simulink model "basicmodel"  (R2018a)
settings: Solver=ode3  StartTime=0.0  StopTime=100  FixedStep=0.1  RelTol=1e-3
InitFcn:
  | data
undefined symbols (not defined in the file or in its folder): sigbuilder_block
libraries: simulink x8
settings Model: Creator=dhruv  LastModifiedBy=dhruv

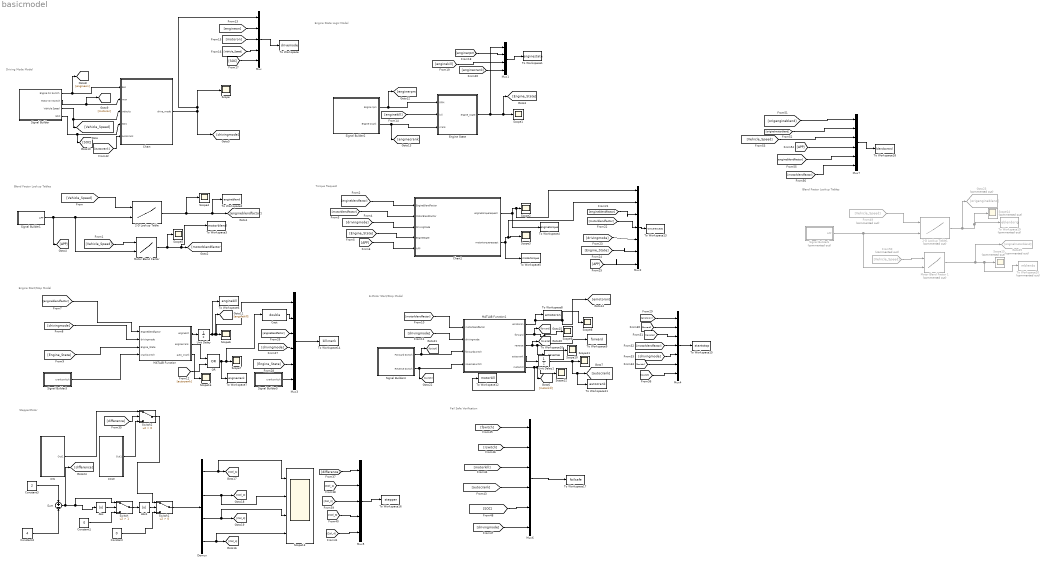
== system basicmodel ==
  note: Fail Safe Verification
  note: E-Motor Start/Stop Model
  note: Engine Start/Stop Model
  note: Torque Request
  note: Engine State Logic Model
  note: Blend Factor Lookup Tables
  note: Driving Mode Model
  note: StepperMotor
  note: Blend Factor Lookup Tables
  2-D Lookup Table : Lookup_n-D  InitFcn=data  BreakpointsForDimension1=Engine_Blend_Factor(2:end,1)  BreakpointsForDimension2=Engine_Blend_Factor(1,2:end)  Table=Engine_Blend_Factor(2:end,2:end)  InternalRulePriority=Speed  RndMeth=Simplest  InputSameDT=on
  2-D Lookup Table1 : Lookup_n-D  Commented=on  InitFcn=data  BreakpointsForDimension1=Engine_Blend_Factoro(2:end,1)  BreakpointsForDimension2=Engine_Blend_Factoro(1,2:end)  Table=Engine_Blend_Factoro(2:end,2:end)  InternalRulePriority=Speed  RndMeth=Simplest  InputSameDT=on
  Abs : Abs
  Abs1 : Abs
  CCW : Subsystem
  CW : Subsystem
  Cast : DataTypeConversion  OutDataTypeStr=double
  Chart : Stateflow chart  TreatAsAtomicUnit=on
  Chart1 : Stateflow chart  TreatAsAtomicUnit=on
  Constant : Constant  Value=0
  Constant1 : Constant  Value=0
  Constant3 : Constant  Value=2
  Constant4 : Constant  Value=4
  Demux : Demux
  "Engine State " : Stateflow chart  TreatAsAtomicUnit=on
  From49 : From  Commented=on  GotoTag=Vehicle_Speed
  From50 : From  Commented=on  GotoTag=Vehicle_Speed
  Goto23 : Goto  Commented=on  GotoTag=origengineblend
  Goto25 : Goto  Commented=on  GotoTag=originalmotorblend
  MATLAB Function : MATLAB Function  TreatAsAtomicUnit=on
  MATLAB Function1 : MATLAB Function  TreatAsAtomicUnit=on
  "Motor Blend Factor " : Lookup_n-D  BreakpointsForDimension1=Motor_Blend_Factor(2:end,1)  BreakpointsForDimension2=Motor_Blend_Factor(1,2:end)  Table=Motor_Blend_Factor(2:end,2:end)  InternalRulePriority=Speed  RndMeth=Simplest  InputSameDT=on
  Motor Blend Factor 1 : Lookup_n-D  Commented=on  BreakpointsForDimension1=Motor_Blend_Factoro(2:end,1)  BreakpointsForDimension2=Motor_Blend_Factoro(1,2:end)  Table=Motor_Blend_Factoro(2:end,2:end)  InternalRulePriority=Speed  RndMeth=Simplest  InputSameDT=on
  Mux : Mux  Inputs=5
  Mux1 : Mux
  Mux2 : Mux  Inputs=7
  Mux3 : Mux  Inputs=6
  Mux4 : Mux  Inputs=7
  Mux5 : Mux  Inputs=5
  Mux6 : Mux  Inputs=6
  Mux7 : Mux  Inputs=6
  OR : Logic  Operator=OR  IconShape=distinctive  AllPortsSameDT=off  OutDataTypeStr=boolean
  Scope{,1..12,16} (14 alike) : Scope
  Scope13 : Scope  NumInputPorts=4
  Scope14 : Scope  Commented=on
  Scope15 : Scope  Commented=on
  Signal Builder : Subsystem  Tag=STV Subsys  LoadFcn=sigbuilder_block('load');  StartFcn=sigbuilder_block('start');  StopFcn=sigbuilder_block('stop');  ClipboardFcn=sigbuilder_block('clipboard');  mask(Sigbuilder block){tuvar=[0:10]}
      mask help: Simulink:masks:SigbuilderBlock_MD
      mask init:
      | if ~strcmp(get_param(bdroot(gcbh),'SimulationStatus'),'stopped') tuvar = sigbuilder_block('maskInit'); end
      settings: CopyFcn=sigbuilder_block('copy');  DeleteFcn=sigbuilder_block('delete');  ModelCloseFcn=sigbuilder_block('modelClose');  PreSaveFcn=sigbuilder_block('preSave');  PauseFcn=sigbuilder_block('pause');  ContinueFcn=sigbuilder_block('continue');  NameChangeFcn=sigbuilder_block('namechange');  OpenFcn=sigbuilder_block('open',[5.5 30 949 418 ]);  CloseFcn=sigbuilder_block('close');
      mask Display: plot(0, 0, 100, 100,[2, 2, 32, 32, 2], [68, 8, 8, 68, 68],[32, 2], [38, 38], [32, 19, 2],[53, 60, 44], [32, 17, 17, 2],[16, 16, 31, 31]);txt = getActiveGroup(gcbh);text(2, 100, txt,'verticalAlignment', 'top');
  Signal Builder1 : Subsystem  Tag=STV Subsys  LoadFcn=sigbuilder_block('load');  StartFcn=sigbuilder_block('start');  StopFcn=sigbuilder_block('stop');  ClipboardFcn=sigbuilder_block('clipboard');  mask(Sigbuilder block){tuvar=[0:10]}
      mask help: Simulink:masks:SigbuilderBlock_MD
      mask init:
      | if ~strcmp(get_param(bdroot(gcbh),'SimulationStatus'),'stopped') tuvar = sigbuilder_block('maskInit'); end
      settings: CopyFcn=sigbuilder_block('copy');  DeleteFcn=sigbuilder_block('delete');  ModelCloseFcn=sigbuilder_block('modelClose');  PreSaveFcn=sigbuilder_block('preSave');  PauseFcn=sigbuilder_block('pause');  ContinueFcn=sigbuilder_block('continue');  NameChangeFcn=sigbuilder_block('namechange');  OpenFcn=sigbuilder_block('open',[267 99 550.5 362.5 ]);  CloseFcn=sigbuilder_block('close');
      mask Display: plot(0, 0, 100, 100,[2, 2, 32, 32, 2], [68, 8, 8, 68, 68],[32, 2], [38, 38], [32, 19, 2],[53, 60, 44], [32, 17, 17, 2],[16, 16, 31, 31]);txt = getActiveGroup(gcbh);text(2, 100, txt,'verticalAlignment', 'top');
  Signal Builder2 : Subsystem  Tag=STV Subsys  LoadFcn=sigbuilder_block('load');  StartFcn=sigbuilder_block('start');  StopFcn=sigbuilder_block('stop');  ClipboardFcn=sigbuilder_block('clipboard');  mask(Sigbuilder block){tuvar=[0:10]}
      mask help: Simulink:masks:SigbuilderBlock_MD
      mask init:
      | if ~strcmp(get_param(bdroot(gcbh),'SimulationStatus'),'stopped') tuvar = sigbuilder_block('maskInit'); end
      settings: CopyFcn=sigbuilder_block('copy');  DeleteFcn=sigbuilder_block('delete');  ModelCloseFcn=sigbuilder_block('modelClose');  PreSaveFcn=sigbuilder_block('preSave');  PauseFcn=sigbuilder_block('pause');  ContinueFcn=sigbuilder_block('continue');  NameChangeFcn=sigbuilder_block('namechange');  OpenFcn=sigbuilder_block('open',[5.5 30 949 418 ]);  CloseFcn=sigbuilder_block('close');
      mask Display: plot(0, 0, 100, 100,[2, 2, 32, 32, 2], [68, 8, 8, 68, 68],[32, 2], [38, 38], [32, 19, 2],[53, 60, 44], [32, 17, 17, 2],[16, 16, 31, 31]);txt = getActiveGroup(gcbh);text(2, 100, txt,'verticalAlignment', 'top');
  Signal Builder3 : Subsystem  Tag=STV Subsys  LoadFcn=sigbuilder_block('load');  StartFcn=sigbuilder_block('start');  StopFcn=sigbuilder_block('stop');  ClipboardFcn=sigbuilder_block('clipboard');  mask(Sigbuilder block){tuvar=[0:10]}
      mask help: Simulink:masks:SigbuilderBlock_MD
      mask init:
      | if ~strcmp(get_param(bdroot(gcbh),'SimulationStatus'),'stopped') tuvar = sigbuilder_block('maskInit'); end
      settings: CopyFcn=sigbuilder_block('copy');  DeleteFcn=sigbuilder_block('delete');  ModelCloseFcn=sigbuilder_block('modelClose');  PreSaveFcn=sigbuilder_block('preSave');  PauseFcn=sigbuilder_block('pause');  ContinueFcn=sigbuilder_block('continue');  NameChangeFcn=sigbuilder_block('namechange');  OpenFcn=sigbuilder_block('open',[404 117.5 550.5 362.5 ]);  CloseFcn=sigbuilder_block('close');
      mask Display: plot(0, 0, 100, 100,[2, 2, 32, 32, 2], [68, 8, 8, 68, 68],[32, 2], [38, 38], [32, 19, 2],[53, 60, 44], [32, 17, 17, 2],[16, 16, 31, 31]);txt = getActiveGroup(gcbh);text(2, 100, txt,'verticalAlignment', 'top');
  Signal Builder4 : Subsystem  Tag=STV Subsys  LoadFcn=sigbuilder_block('load');  StartFcn=sigbuilder_block('start');  StopFcn=sigbuilder_block('stop');  ClipboardFcn=sigbuilder_block('clipboard');  mask(Sigbuilder block){tuvar=[0:10]}
      mask help: Simulink:masks:SigbuilderBlock_MD
      mask init:
      | if ~strcmp(get_param(bdroot(gcbh),'SimulationStatus'),'stopped') tuvar = sigbuilder_block('maskInit'); end
      settings: CopyFcn=sigbuilder_block('copy');  DeleteFcn=sigbuilder_block('delete');  ModelCloseFcn=sigbuilder_block('modelClose');  PreSaveFcn=sigbuilder_block('preSave');  PauseFcn=sigbuilder_block('pause');  ContinueFcn=sigbuilder_block('continue');  NameChangeFcn=sigbuilder_block('namechange');  OpenFcn=sigbuilder_block('open',[404 117.5 550.5 362.5 ]);  CloseFcn=sigbuilder_block('close');
      mask Display: plot(0, 0, 100, 100,[2, 2, 32, 32, 2], [68, 8, 8, 68, 68],[32, 2], [38, 38], [32, 19, 2],[53, 60, 44], [32, 17, 17, 2],[16, 16, 31, 31]);txt = getActiveGroup(gcbh);text(2, 100, txt,'verticalAlignment', 'top');
  Signal Builder5 : Subsystem  Tag=STV Subsys  LoadFcn=sigbuilder_block('load');  StartFcn=sigbuilder_block('start');  StopFcn=sigbuilder_block('stop');  ClipboardFcn=sigbuilder_block('clipboard');  mask(Sigbuilder block){tuvar=[0:10]}
      mask help: Simulink:masks:SigbuilderBlock_MD
      mask init:
      | if ~strcmp(get_param(bdroot(gcbh),'SimulationStatus'),'stopped') tuvar = sigbuilder_block('maskInit'); end
      settings: CopyFcn=sigbuilder_block('copy');  DeleteFcn=sigbuilder_block('delete');  ModelCloseFcn=sigbuilder_block('modelClose');  PreSaveFcn=sigbuilder_block('preSave');  PauseFcn=sigbuilder_block('pause');  ContinueFcn=sigbuilder_block('continue');  NameChangeFcn=sigbuilder_block('namechange');  OpenFcn=sigbuilder_block('open',[404 117.5 550.5 362.5 ]);  CloseFcn=sigbuilder_block('close');
      mask Display: plot(0, 0, 100, 100,[2, 2, 32, 32, 2], [68, 8, 8, 68, 68],[32, 2], [38, 38], [32, 19, 2],[53, 60, 44], [32, 17, 17, 2],[16, 16, 31, 31]);txt = getActiveGroup(gcbh);text(2, 100, txt,'verticalAlignment', 'top');
  Signal Builder6 : Subsystem  Tag=STV Subsys  Commented=on  LoadFcn=sigbuilder_block('load');  StartFcn=sigbuilder_block('start');  StopFcn=sigbuilder_block('stop');  ClipboardFcn=sigbuilder_block('clipboard');  mask(Sigbuilder block){tuvar=[0:10]}
      mask help: Simulink:masks:SigbuilderBlock_MD
      mask init:
      | if ~strcmp(get_param(bdroot(gcbh),'SimulationStatus'),'stopped') tuvar = sigbuilder_block('maskInit'); end
      settings: CopyFcn=sigbuilder_block('copy');  DeleteFcn=sigbuilder_block('delete');  ModelCloseFcn=sigbuilder_block('modelClose');  PreSaveFcn=sigbuilder_block('preSave');  PauseFcn=sigbuilder_block('pause');  ContinueFcn=sigbuilder_block('continue');  NameChangeFcn=sigbuilder_block('namechange');  OpenFcn=sigbuilder_block('open',[267 99 550.5 362.5 ]);  CloseFcn=sigbuilder_block('close');
      mask Display: plot(0, 0, 100, 100,[2, 2, 32, 32, 2], [68, 8, 8, 68, 68],[32, 2], [38, 38], [32, 19, 2],[53, 60, 44], [32, 17, 17, 2],[16, 16, 31, 31]);txt = getActiveGroup(gcbh);text(2, 100, txt,'verticalAlignment', 'top');
  Sum : Sum  Inputs=+-
  Switch : Switch  Criteria=u2 > Threshold  Threshold=1
  Switch1 : Switch  Criteria=u2 > Threshold
  Switch2 : Switch  Criteria=u2 > Threshold
  To Workspace : ToWorkspace  VariableName=drivemode  SaveFormat=Timeseries  SampleTime=-1
  To Workspace1 : ToWorkspace  VariableName=enginestate  SaveFormat=Timeseries  SampleTime=-1
  To Workspace10 : ToWorkspace  VariableName=reverse  SaveFormat=Timeseries  SampleTime=-1
  To Workspace11 : ToWorkspace  VariableName=autocrank  SaveFormat=Timeseries  SampleTime=-1
  To Workspace12 : ToWorkspace  VariableName=motorkill  SaveFormat=Timeseries  SampleTime=-1
  To Workspace13 : ToWorkspace  VariableName=torquerequests  SaveFormat=Timeseries  SampleTime=-1
  To Workspace14 : ToWorkspace  VariableName=killcrank  SaveFormat=Timeseries  SampleTime=-1
  To Workspace15 : ToWorkspace  VariableName=startstop  SaveFormat=Timeseries  SampleTime=-1
  To Workspace16 : ToWorkspace  VariableName=stepper  SaveFormat=Timeseries  SampleTime=-1
  To Workspace17 : ToWorkspace  VariableName=failsafe  SaveFormat=Timeseries  SampleTime=-1
  To Workspace18 : ToWorkspace  VariableName=blendcontrol  SaveFormat=Timeseries  SampleTime=-1
  To Workspace19 : ToWorkspace  Commented=on  VariableName=eblendorig  SaveFormat=Timeseries  SampleTime=-1
  To Workspace2 : ToWorkspace  VariableName=engineblend  SaveFormat=Timeseries  SampleTime=-1
  To Workspace20 : ToWorkspace  Commented=on  VariableName=mblendo  SaveFormat=Timeseries  SampleTime=-1
  To Workspace3 : ToWorkspace  VariableName=motorblend  SaveFormat=Timeseries  SampleTime=-1
  To Workspace4 : ToWorkspace  VariableName=enginetorque  SaveFormat=Timeseries  SampleTime=-1
  To Workspace5 : ToWorkspace  VariableName=motortorque  SaveFormat=Timeseries  SampleTime=-1
  To Workspace6 : ToWorkspace  VariableName=enginekill  SaveFormat=Timeseries  SampleTime=-1
  To Workspace7 : ToWorkspace  VariableName=enginecrank  SaveFormat=Timeseries  SampleTime=-1
  To Workspace8 : ToWorkspace  VariableName=emotoron  SaveFormat=Timeseries  SampleTime=-1
  To Workspace9 : ToWorkspace  VariableName=forward  SaveFormat=Timeseries  SampleTime=-1
  Unit Delay : UnitDelay  SampleTime=-1
  Unit Delay1 : UnitDelay  SampleTime=-1
  wires:
  Signal Builder/2(Motor On Switch) -> [motoron], Chart/2(mon)
  Signal Builder/1(Engine On Switch) -> [engineon], Chart/1(Eon)
  Signal Builder/3(Vehicle Speed) -> [Vehicle_Speed], Chart/3(velocity)
  Signal Builder1/1(APP) -> [APP], "Motor Blend Factor "/2, 2-D Lookup Table/2
  [Vehicle_Speed] -> 2-D Lookup Table/1
  [Vehicle_Speed] -> "Motor Blend Factor "/1
  2-D Lookup Table/1 -> Scope4/1, To Workspace2/1, [engineblendfactor]
  "Motor Blend Factor "/1 -> Scope5/1, To Workspace3/1, [motorblendfactor]
  Chart/1(drive_mode) -> Mux/1, Scope/1, [drivingmode]
  Signal Builder2/1(Engine rpm) -> [enginerpm], "Engine State "/1(RPM)
  [engineblendfactor] -> Chart1/1(EngineBlendFactor)
  [motorblendfactor] -> Chart1/2(MotorBlendFactor)
  [drivingmode] -> Chart1/3(DrivingMode)
  [Engine_State] -> Chart1/4(EngineState)
  [APP] -> Chart1/5(APP)
  Chart1/1(enginetorquerequest) -> Mux2/1, Scope2/1, To Workspace4/1
  Chart1/2(motortorquerequest) -> Mux2/2, Scope3/1, To Workspace5/1
  [engineblendfactor] -> MATLAB Function/1(engineblendfactor)
  [drivingmode] -> MATLAB Function/2(drivingmode)
  [Engine_State] -> MATLAB Function/3(Engine_State)
  Signal Builder3/1(crankswitch) -> MATLAB Function/4(crankswitch)
  MATLAB Function/2(enginecrank) -> OR/1
  [motorblendfactor] -> MATLAB Function1/1(motorblendfactor)
  [drivingmode] -> MATLAB Function1/2(drivingmode)
  Signal Builder4/1(Forward Switch) -> [fswitch], MATLAB Function1/3(forwardswitch)
  Signal Builder4/2(Reverse Switch) -> [rswitch], MATLAB Function1/4(reverseswitch)
  MATLAB Function1/1(emotoron) -> To Workspace8/1, [emotoron], Scope8/1
  MATLAB Function1/3(reverse) -> [reverse], To Workspace10/1, Scope10/1
  [enginekill] -> "Engine State "/2(kill)
  MATLAB Function/1(enginekill) -> Unit Delay/1
  "Engine State "/1(engine_state) -> Mux1/1, [Engine_State], Scope1/1
  Unit Delay/1 -> To Workspace6/1, [enginekill], Mux3/1, Scope6/1
  MATLAB Function1/2(forward) -> [forward], To Workspace9/1, Scope9/1
  MATLAB Function1/4(autocrank) -> Unit Delay1/1
  MATLAB Function1/5(motorkill) -> To Workspace12/1, [motorkill], Scope12/1
  [difference] -> Switch2/2
  CCW/1(Out1) -> Switch2/3
  CW/1(Out1) -> Switch2/1
  Constant3/1 -> Sum/1
  Demux/4 -> Scope13/4, [Coil_4]
  Constant4/1 -> Sum/2
  Demux/1 -> Scope13/1, [Coil_1]
  Demux/2 -> Scope13/2, [Coil_2]
  Sum/1 -> [difference], Switch/1, Abs/1
  Demux/3 -> Scope13/3, [Coil_3]
  Abs/1 -> Switch/2
  [autocrank] -> OR/2
  OR/1 -> To Workspace7/1, Cast/1, Scope7/1
  Switch/1 -> Abs1/1
  Switch2/1 -> Switch1/1
  Constant/1 -> Switch1/3
  Switch1/1 -> Demux/1
  Constant1/1 -> Switch/3
  Abs1/1 -> Switch1/2
  Signal Builder/4(SOC) -> [SOC], Chart/4(SOC)
  [engineon] -> Mux/2
  [motoron] -> Mux/3
  [Vehicle_Speed] -> Mux/4
  [SOC] -> Mux/5
  Mux/1 -> To Workspace/1
  Signal Builder2/2(Engine Crank) -> [enginecrank], "Engine State "/3(crank)
  Mux1/1 -> To Workspace1/1
  [enginerpm] -> Mux1/2
  [enginekill] -> Mux1/3
  [enginecrank] -> Mux1/4
  [engineblendfactor] -> Mux2/3
  [motorblendfactor] -> Mux2/4
  [drivingmode] -> Mux2/5
  [Engine_State] -> Mux2/6
  [APP] -> Mux2/7
  Mux2/1 -> To Workspace13/1
  [engineblendfactor] -> Mux3/3
  [drivingmode] -> Mux3/4
  [Engine_State] -> Mux3/5
  Signal Builder5/1(crankswitch) -> Mux3/6
  Mux3/1 -> To Workspace14/1
  [emotoron] -> Mux4/1
  [forward] -> Mux4/2
  [reverse] -> Mux4/3
  [motorblendfactor] -> Mux4/4
  [drivingmode] -> Mux4/5
  [fswitch] -> Mux4/6
  [rswitch] -> Mux4/7
  Mux4/1 -> To Workspace15/1
  [difference] -> Mux5/1
  [Coil_1] -> Mux5/2
  [Coil_2] -> Mux5/3
  [Coil_3] -> Mux5/4
  [Coil_4] -> Mux5/5
  Mux5/1 -> To Workspace16/1
  Cast/1 -> Mux3/2
  [autocrank] -> Chart/5(autocrank)
  Unit Delay1/1 -> To Workspace11/1, [autocrank], Scope11/1
  [fswitch] -> Mux6/1
  [rswitch] -> Mux6/2
  [motorkill] -> Mux6/3
  [autocrank] -> Mux6/4
  [drivingmode] -> Mux6/6
  [SOC] -> Mux6/5
  Mux6/1 -> To Workspace17/1
  Signal Builder6/1(APP) -> Motor Blend Factor 1/2, 2-D Lookup Table1/2
  From49/1 -> 2-D Lookup Table1/1
  Motor Blend Factor 1/1 -> Goto25/1, To Workspace20/1, Scope15/1
  From50/1 -> Motor Blend Factor 1/1
  2-D Lookup Table1/1 -> Goto23/1, To Workspace19/1, Scope14/1
  [origengineblend] -> Mux7/1
  [originalmotorblend] -> Mux7/2
  [Vehicle_Speed] -> Mux7/3
  [APP] -> Mux7/4
  [engineblendfactor] -> Mux7/5
  [motorblendfactor] -> Mux7/6
  Mux7/1 -> To Workspace18/1
  MATLAB Function/3(auto_crank) -> Scope16/1

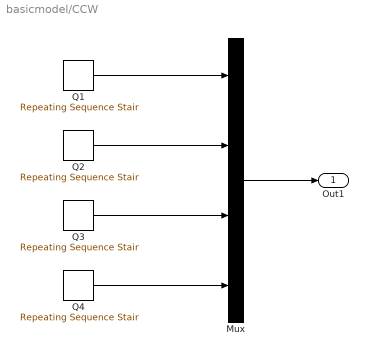
== system basicmodel/CCW ==
  Mux : Mux
  Q1 : simulink/Sources/Repeating Sequence Stair  OutValues=[1 0 0 0 0 0 1 1 1].'  tsamp=-1  OutMin=[]  OutMax=[]  OutDataTypeStr=double  OutputDataTypeScalingMode=double  OutDataType=fixdt(0,8)  ConRadixGroup=Best Precision: Vector-wise  OutScaling=2^-12
  Q2 : simulink/Sources/Repeating Sequence Stair  OutValues=[0 0 1 1 1 0 0 0 0].'  tsamp=-1  OutMin=[]  OutMax=[]  OutDataTypeStr=double  OutputDataTypeScalingMode=double  OutDataType=fixdt(0,8)  ConRadixGroup=Best Precision: Vector-wise  OutScaling=2^-12
  Q3 : simulink/Sources/Repeating Sequence Stair  OutValues=[1 1 1 0 0 0 0 0 1].'  tsamp=-1  OutMin=[]  OutMax=[]  OutDataTypeStr=double  OutputDataTypeScalingMode=double  OutDataType=fixdt(0,8)  ConRadixGroup=Best Precision: Vector-wise  OutScaling=2^-12
  Q4 : simulink/Sources/Repeating Sequence Stair  OutValues=[0 0 0 0 1 1 1 0 0].'  tsamp=-1  OutMin=[]  OutMax=[]  OutDataTypeStr=double  OutputDataTypeScalingMode=double  OutDataType=fixdt(0,8)  ConRadixGroup=Best Precision: Vector-wise  OutScaling=2^-12
  Out1 : Outport
  wires:
  Q1/1 -> Mux/1
  Q2/1 -> Mux/2
  Q3/1 -> Mux/3
  Q4/1 -> Mux/4
  Mux/1 -> Out1/1

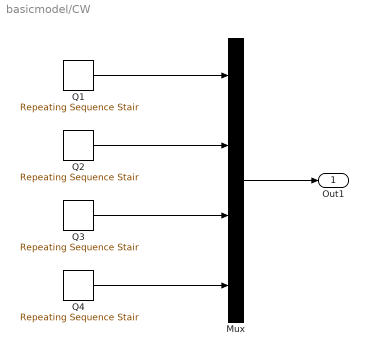
== system basicmodel/CW ==
  Mux : Mux
  Q1 : simulink/Sources/Repeating Sequence Stair  OutValues=[1 1 1 0 0 0 0 0 1].'  tsamp=-1  OutMin=[]  OutMax=[]  OutDataTypeStr=double  OutputDataTypeScalingMode=double  OutDataType=fixdt(0,8)  ConRadixGroup=Best Precision: Vector-wise  OutScaling=2^-12
  Q2 : simulink/Sources/Repeating Sequence Stair  OutValues=[0 0 0 0 1 1 1 0 0].'  tsamp=-1  OutMin=[]  OutMax=[]  OutDataTypeStr=double  OutputDataTypeScalingMode=double  OutDataType=fixdt(0,8)  ConRadixGroup=Best Precision: Vector-wise  OutScaling=2^-12
  Q3 : simulink/Sources/Repeating Sequence Stair  OutValues=[1 0 0 0 0 0 1 1 1].'  tsamp=-1  OutMin=[]  OutMax=[]  OutDataTypeStr=double  OutputDataTypeScalingMode=double  OutDataType=fixdt(0,8)  ConRadixGroup=Best Precision: Vector-wise  OutScaling=2^-12
  Q4 : simulink/Sources/Repeating Sequence Stair  OutValues=[0 0 1 1 1 0 0 0 0].'  tsamp=-1  OutMin=[]  OutMax=[]  OutDataTypeStr=double  OutputDataTypeScalingMode=double  OutDataType=fixdt(0,8)  ConRadixGroup=Best Precision: Vector-wise  OutScaling=2^-12
  Out1 : Outport
  wires:
  Mux/1 -> Out1/1
  Q4/1 -> Mux/4
  Q3/1 -> Mux/3
  Q2/1 -> Mux/2
  Q1/1 -> Mux/1

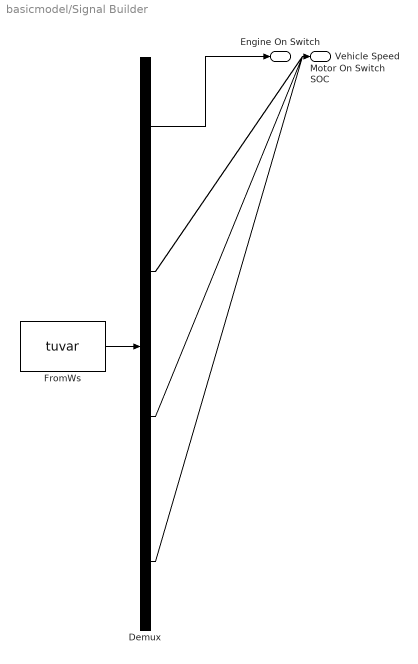
== system basicmodel/Signal Builder ==
  Demux : Demux  Tag=STV Demux
  FromWs : FromWorkspace  Tag=STV FromWs  VariableName=tuvar  SampleTime=0
      SigBuilderData=|
      | common.afterFinalStr = 'Extrapolate'
      | common.sampleTime = 0
      | dataSet.timeRange = [0 100]
      | dataSet.name = 'Group 1'
      | sbobj.Groups.Name = 'Group 1'
      | sbobj.Groups.Signals(1).Name = 'Engine On Switch'
      | sbobj.Groups.Signals(1).XData = [0 33.7 33.7 40.9 40.9 51.4 51.4 59 59 88.6 88.6 94 94 100]
      | sbobj.Groups.Signals(1).YData = [0 0 1 1 0 0 1 1 0 0 1 1 0 0]
      | sbobj.Groups.Signals(2).Name = 'Motor On Switch'
      | sbobj.Groups.Signals(2).XData = [0 5 5 30.2 30.2 48.6 48.6 65 65 80.4 80.4 85.8 85.8 100]
      | sbobj.Groups.Signals(2).YData = [0 0 1 1 0 0 1 1 0 0 1 1 0 0]
      | sbobj.Groups.Signals(3).Name = 'Vehicle Speed'
      | sbobj.Groups.Signals(3).XData = [0 4 4 12.1 12.1 46.2 57.6 74.7 74.7 89.8 100]
      | sbobj.Groups.Signals(3).YData = [0 0 0.6 1.4 10 0.4 0.6 9.9 10.2 0.8 5.2]
      | sbobj.Groups.Signals(4).Name = 'SOC'
      | sbobj.Groups.Signals(4).XData = [0 0.9 0.9 9.2 27 27 42.3 42.3 46.4 46.4 52.9 52.9 63 63 100]
      | sbobj.Groups.Signals(4).YData = [0 0 0.9 0.9 0.7 2.34 1.86 1.9 1.95 2.6 2.65 1.9 1.95 2.55 2.8]
      | sbobj.Groups.TimeRange = [0 100]
  Engine On Switch : Outport  Tag=STV Outport
  Motor On Switch : Outport  Tag=STV Outport  Port=2
  Vehicle Speed : Outport  Tag=STV Outport  Port=3
  SOC : Outport  Tag=STV Outport  Port=4
  wires:
  Demux/1 -> Engine On Switch/1
  FromWs/1 -> Demux/1
  Demux/2 -> Motor On Switch/1
  Demux/3 -> Vehicle Speed/1
  Demux/4 -> SOC/1

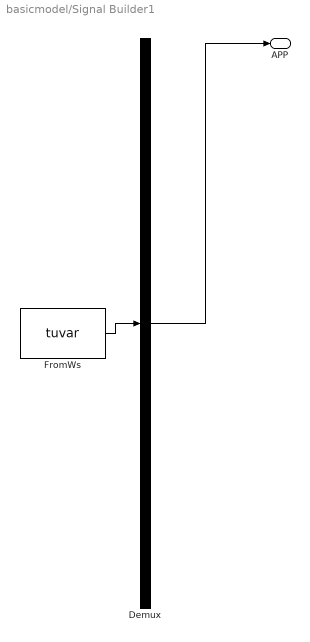
== system basicmodel/Signal Builder1 ==
  Demux : Demux  Tag=STV Demux  Outputs=1
  FromWs : FromWorkspace  Tag=STV FromWs  VariableName=tuvar  SampleTime=0
      SigBuilderData=|
      | common.afterFinalStr = 'Extrapolate'
      | common.sampleTime = 0
      | dataSet.timeRange = [0 100]
      | dataSet.name = 'Group 1'
      | sbobj.Groups.Name = 'Group 1'
      | sbobj.Groups.Signals.Name = 'APP'
      | sbobj.Groups.Signals.XData = [0 0.6 0.6 6 6 12.1 12.1 20.8 20.8 44.1 44.1 49.6 49.6 73 73 100]
      | sbobj.Groups.Signals.YData = [0 0 12.6 12.6 0 0 10 10 5.2 5 12.2 12.2 0 0 23.6 23.6]
      | sbobj.Groups.TimeRange = [0 100]
  APP : Outport  Tag=STV Outport
  wires:
  Demux/1 -> APP/1
  FromWs/1 -> Demux/1

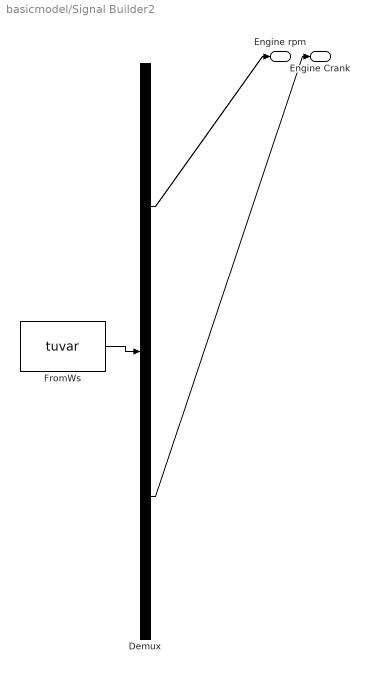
== system basicmodel/Signal Builder2 ==
  Demux : Demux  Tag=STV Demux  Outputs=2
  FromWs : FromWorkspace  Tag=STV FromWs  VariableName=tuvar  SampleTime=0
      SigBuilderData=|
      | common.afterFinalStr = 'Extrapolate'
      | common.sampleTime = 0
      | dataSet.timeRange = [0 100]
      | dataSet.name = 'Group 1'
      | sbobj.Groups.Name = 'Group 1'
      | sbobj.Groups.Signals(1).Name = 'Engine rpm'
      | sbobj.Groups.Signals(1).XData = [0 14.4 14.4 78.3 78.3 89 89 92.1 92.1 97.6 97.6 100]
      | sbobj.Groups.Signals(1).YData = [0 0 900 900 500 500 820 820 800 800 0 0]
      | sbobj.Groups.Signals(2).Name = 'Engine Crank'
      | sbobj.Groups.Signals(2).XData = [0 11.6 11.6 16.1 16.1 48.6 60.2 84.1 84.1 95 95 100]
      | sbobj.Groups.Signals(2).YData = [0 0 1 1 0 0 0 0 1 1 0 0]
      | sbobj.Groups.TimeRange = [0 100]
  Engine rpm : Outport  Tag=STV Outport
  Engine Crank : Outport  Tag=STV Outport  Port=2
  wires:
  FromWs/1 -> Demux/1
  Demux/1 -> Engine rpm/1
  Demux/2 -> Engine Crank/1

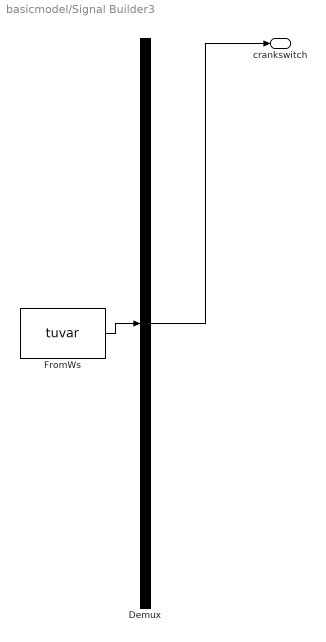
== system basicmodel/Signal Builder3 ==
  Demux : Demux  Tag=STV Demux  Outputs=1
  FromWs : FromWorkspace  Tag=STV FromWs  VariableName=tuvar  SampleTime=0
      SigBuilderData=|
      | common.afterFinalStr = 'Extrapolate'
      | common.sampleTime = 0
      | dataSet.timeRange = [0 100]
      | dataSet.name = 'Group 1'
      | sbobj.Groups.Name = 'Group 1'
      | sbobj.Groups.Signals.Name = 'crankswitch'
      | sbobj.Groups.Signals.XData = [0 24.6 24.6 35.4 35.4 100]
      | sbobj.Groups.Signals.YData = [0 0 1 1 0 0]
      | sbobj.Groups.TimeRange = [0 100]
  crankswitch : Outport  Tag=STV Outport
  wires:
  Demux/1 -> crankswitch/1
  FromWs/1 -> Demux/1

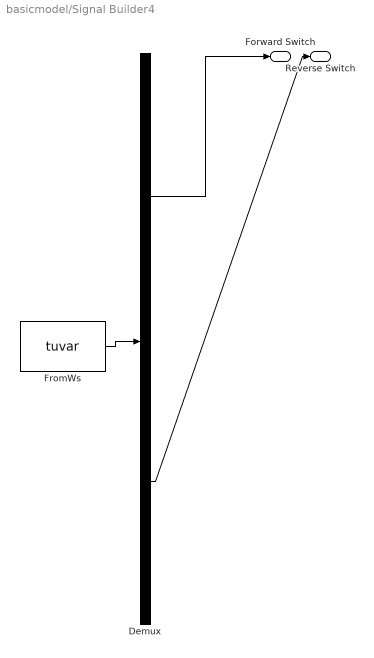
== system basicmodel/Signal Builder4 ==
  Demux : Demux  Tag=STV Demux  Outputs=2
  FromWs : FromWorkspace  Tag=STV FromWs  VariableName=tuvar  SampleTime=0
      SigBuilderData=|
      | common.afterFinalStr = 'Extrapolate'
      | common.sampleTime = 0
      | dataSet.timeRange = [0 100]
      | dataSet.name = 'Group 1'
      | sbobj.Groups.Name = 'Group 1'
      | sbobj.Groups.Signals(1).Name = 'Forward Switch'
      | sbobj.Groups.Signals(1).XData = [0 20.6 20.6 30.2 30.2 100]
      | sbobj.Groups.Signals(1).YData = [0 0 1 1 0 0]
      | sbobj.Groups.Signals(2).Name = 'Reverse Switch'
      | sbobj.Groups.Signals(2).XData = [0 38.4 38.4 46.4 46.4 100]
      | sbobj.Groups.Signals(2).YData = [0 0 1 1 0 0]
      | sbobj.Groups.TimeRange = [0 100]
  Forward Switch : Outport  Tag=STV Outport
  Reverse Switch : Outport  Tag=STV Outport  Port=2
  wires:
  Demux/1 -> Forward Switch/1
  FromWs/1 -> Demux/1
  Demux/2 -> Reverse Switch/1

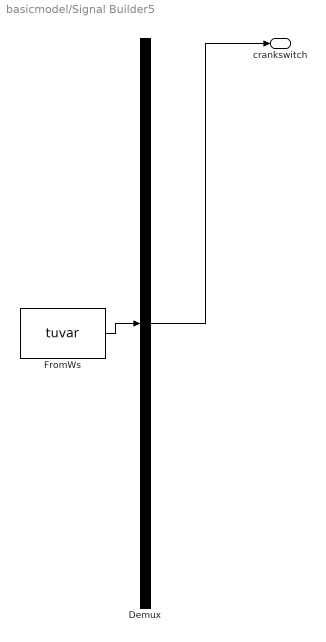
== system basicmodel/Signal Builder5 ==
  Demux : Demux  Tag=STV Demux  Outputs=1
  FromWs : FromWorkspace  Tag=STV FromWs  VariableName=tuvar  SampleTime=0
      SigBuilderData=|
      | common.afterFinalStr = 'Extrapolate'
      | common.sampleTime = 0
      | dataSet.timeRange = [0 100]
      | dataSet.name = 'Group 1'
      | sbobj.Groups.Name = 'Group 1'
      | sbobj.Groups.Signals.Name = 'crankswitch'
      | sbobj.Groups.Signals.XData = [0 24.6 24.6 35.4 35.4 100]
      | sbobj.Groups.Signals.YData = [0 0 1 1 0 0]
      | sbobj.Groups.TimeRange = [0 100]
  crankswitch : Outport  Tag=STV Outport
  wires:
  Demux/1 -> crankswitch/1
  FromWs/1 -> Demux/1

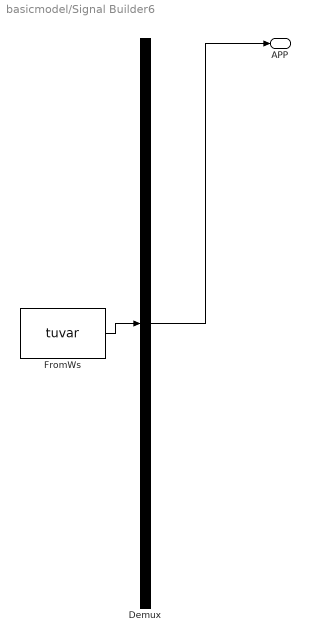
== system basicmodel/Signal Builder6 ==
  Demux : Demux  Tag=STV Demux  Outputs=1
  FromWs : FromWorkspace  Tag=STV FromWs  VariableName=tuvar  SampleTime=0
      SigBuilderData=|
      | common.afterFinalStr = 'Extrapolate'
      | common.sampleTime = 0
      | dataSet.timeRange = [0 100]
      | dataSet.name = 'Group 1'
      | sbobj.Groups.Name = 'Group 1'
      | sbobj.Groups.Signals.Name = 'APP'
      | sbobj.Groups.Signals.XData = [0 0.6 0.6 6 6 12.1 12.1 20.8 20.8 44.1 44.1 49.6 49.6 73 73 100]
      | sbobj.Groups.Signals.YData = [0 0 12.6 12.6 0 0 10 10 5.2 5 12.2 12.2 0 0 23.6 23.6]
      | sbobj.Groups.TimeRange = [0 100]
  APP : Outport  Tag=STV Outport
  wires:
  Demux/1 -> APP/1
  FromWs/1 -> Demux/1

== stateflow chart basicmodel/Engine State  ==
  state Engine_State_Logic
    state Engineoffstate
      during:
      engine_state=1;
    state EngineCrankState
      during:
      engine_state=2;
    state EngineWarmUp
      during:
      engine_state=3;
    state EngineOn
      during:
      engine_state=4;
    state EngineStartFail
      entry:
      engine_state=5;
    (default) -> Engineoffstate
    Engineoffstate -> EngineCrankState : [crank ==1 && kill==0]
    EngineStartFail -> Engineoffstate
    EngineOn -> Engineoffstate : [RPM<50 || kill==1]
    EngineCrankState -> EngineWarmUp [order 1] : [RPM>800 && after(0.6,sec)]
    EngineCrankState -> EngineStartFail [order 2] : [RPM<=800 && after(1,sec)]
    EngineWarmUp -> EngineOn [order 1] : [RPM>=500 && after(1,sec)]
    EngineWarmUp -> EngineStartFail [order 2] : [RPM<500 && after(1,sec)]
  (default) -> Engine_State_Logic
  data: RPM input; kill input; crank input; engine_state output

== stateflow chart basicmodel/Chart1 ==
  state ThrottleRequest
    state intermediate
      during:
      enginetorquerequest=7.5;
    state Engine_Solo
      during:
      enginetorquerequest=APP;
      motortorquerequest=0;
    state Blending
      during:
      enginetorquerequest=APP*EngineBlendFactor;
      motortorquerequest=APP*MotorBlendFactor;
    state Electric_Solo
      during:
      motortorquerequest=APP;
      enginetorquerequest=0;
    intermediate -> Blending [order 1] : [EngineState==4 && DrivingMode==2]
    Engine_Solo -> intermediate [order 1] : [EngineState==2 || EngineState==3 && DrivingMode==2 ]
    intermediate -> Engine_Solo [order 2] : [DrivingMode==3]
    Blending -> intermediate [order 1] : [EngineState==2 || EngineState==3 && DrivingMode==2]
    Engine_Solo -> Blending [order 2] : [EngineState==4 && DrivingMode==2]
    Engine_Solo -> Electric_Solo [order 3] : [DrivingMode==1]
    Electric_Solo -> Engine_Solo [order 1] : [DrivingMode==3]
    Blending -> Engine_Solo [order 3] : [DrivingMode==3]
    Electric_Solo -> Blending [order 2] : [DrivingMode==2]
    Blending -> Electric_Solo [order 2] : [DrivingMode==1]
    (default) -> Electric_Solo
  (default) -> ThrottleRequest
  data: EngineBlendFactor input; MotorBlendFactor input; DrivingMode input; EngineState input; APP input; enginetorquerequest output; motortorquerequest output

== stateflow chart basicmodel/Chart ==
  state Driving_Mode_Model
    state Electric_Solo
      entry:
      drive_mode=1;
    state Engine_Solo
      during:
      drive_mode=3;
    state Blending_Mode
      during:
      drive_mode=2;
    Electric_Solo -> Engine_Solo [order 2] : [velocity<1 && Eon==1 && mon==0 || SOC<0.3 || autocrank==1]
    Engine_Solo -> Electric_Solo [order 1] : [velocity<1 && Eon==0 && mon==1 && SOC>=0.3]
    Blending_Mode -> Electric_Solo [order 1] : [velocity<1 && Eon==0 && mon==1 && SOC>=0.3]
    Electric_Solo -> Blending_Mode [order 1] : [velocity<1 && Eon==0 && mon==0 && SOC>=0.3]
    Blending_Mode -> Engine_Solo [order 2] : [velocity<1 && Eon==1 && mon==0 || SOC<0.3 || autocrank==1]
    Engine_Solo -> Blending_Mode [order 2] : [velocity<1 && Eon==0 && mon==0 && SOC>=0.3]
  (default) -> Electric_Solo
  data: Eon input; mon input; velocity input; drive_mode output; SOC input; autocrank input

== matlab function basicmodel/MATLAB Function ==
  data: engineblendfactor input; enginekill output; drivingmode input; Engine_State input; crankswitch input; enginecrank output; auto_crank output
function [enginekill, enginecrank,auto_crank] = fcn(engineblendfactor, drivingmode, Engine_State, crankswitch)
if drivingmode==1
    enginekill=1;
elseif drivingmode==2
    if engineblendfactor>0.01
        enginekill=0;
    else
        enginekill=1;
    end
else
    enginekill=0;
end

if drivingmode==1
    manualcrank=0;
    enginecrank=manualcrank;
    auto_crank=0;
elseif drivingmode==2
    if engineblendfactor>0.01 && Engine_State==1
        auto_crank=1;
        enginecrank=auto_crank;
    else
        enginecrank=0;
        auto_crank=0;
    end
elseif drivingmode==3 && crankswitch==1
    manualcrank=1;
    enginecrank=manualcrank;
    auto_crank = 0;
else
    enginecrank=0;
    auto_crank=0;
end
end

== matlab function basicmodel/MATLAB Function1 ==
  data: motorblendfactor input; emotoron output; drivingmode input; forwardswitch input; reverseswitch input; forward output; reverse output; autocrank output; motorkill output
function [emotoron, forward, reverse, autocrank,motorkill] = fcn(motorblendfactor, drivingmode, forwardswitch, reverseswitch)
if drivingmode==1
    emotoron=1;
elseif drivingmode==2
    if motorblendfactor>0.01
        emotoron=1;
    else
        emotoron=0;
    end
else
    emotoron=0;
end

if drivingmode==1
    if forwardswitch==1 && reverseswitch==0
        forward=1;
        reverse=0;
    elseif forwardswitch==0 && reverseswitch==1
        forward=0;
        reverse=1;
    else
        forward=0;
        reverse=0;
    end    
elseif drivingmode==2
        forward=1;
        reverse=0;
else
    forward=0;
    reverse=0;
end    
if reverseswitch==1 && forwardswitch==1
        motorkill=1;
        autocrank=motorkill;
else
        motorkill=0;
        autocrank=0;
end
end
